simulink model "Energy"  (R2014a)
settings: Solver=ode45  StartTime=0.0  StopTime=10.0  RelTol=1e-3
undefined symbols (not defined in the file): nfs
settings Model: Creator=sadidsaze6  LastModifiedBy=sadidsaze6

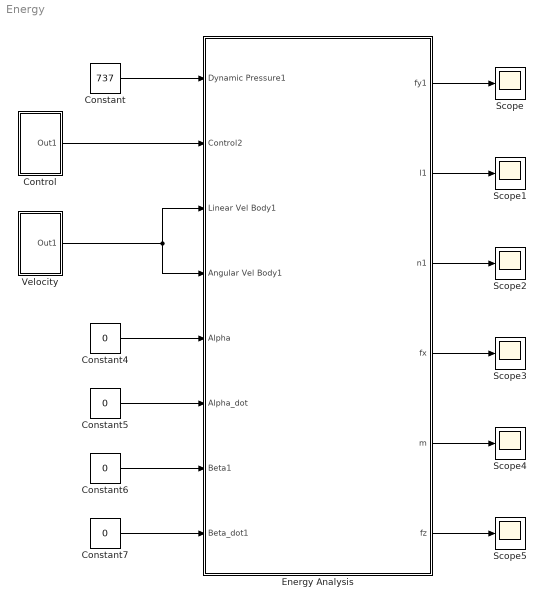
== system Energy ==
  Constant : Constant  Value=737
  Constant{4..7} (4 alike) : Constant  Value=0
  Control : Subsystem
  Energy Analysis : Subsystem  mask{ae=nfs}
      mask prompts: ae "Aero Coefficients"
  Scope{,1..5} (6 alike) : Scope
      Scope2 settings: SaveName=ScopeData2
      Scope3 settings: SaveName=ScopeData3
      Scope4 settings: SaveName=ScopeData4
      Scope5 settings: SaveName=ScopeData5
  Velocity : Subsystem
  wires:
  Constant4/1 -> Energy Analysis/5(Alpha)
  Constant/1 -> Energy Analysis/1(Dynamic Pressure1)
  Constant6/1 -> Energy Analysis/7(Beta1)
  Constant5/1 -> Energy Analysis/6(Alpha_dot)
  Constant7/1 -> Energy Analysis/8(Beta_dot1)
  Energy Analysis/2(l1) -> Scope1/1
  Energy Analysis/1(fy1) -> Scope/1
  Energy Analysis/3(n1) -> Scope2/1
  Energy Analysis/4(fx) -> Scope3/1
  Energy Analysis/5(m) -> Scope4/1
  Energy Analysis/6(fz) -> Scope5/1
  Control/1(Out1) -> Energy Analysis/2(Control2)
  Velocity/1(Out1) -> Energy Analysis/4(Angular Vel Body1), Energy Analysis/3(Linear Vel Body1)

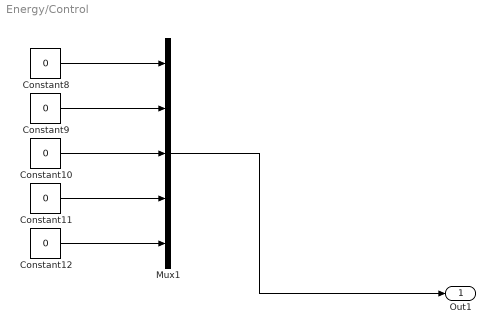
== system Energy/Control ==
  Constant{8..12} (5 alike) : Constant  Value=0
  Mux1 : Mux  Inputs=5
  Out1 : Outport
  wires:
  Mux1/1 -> Out1/1
  Constant10/1 -> Mux1/3
  Constant9/1 -> Mux1/2
  Constant8/1 -> Mux1/1
  Constant11/1 -> Mux1/4
  Constant12/1 -> Mux1/5

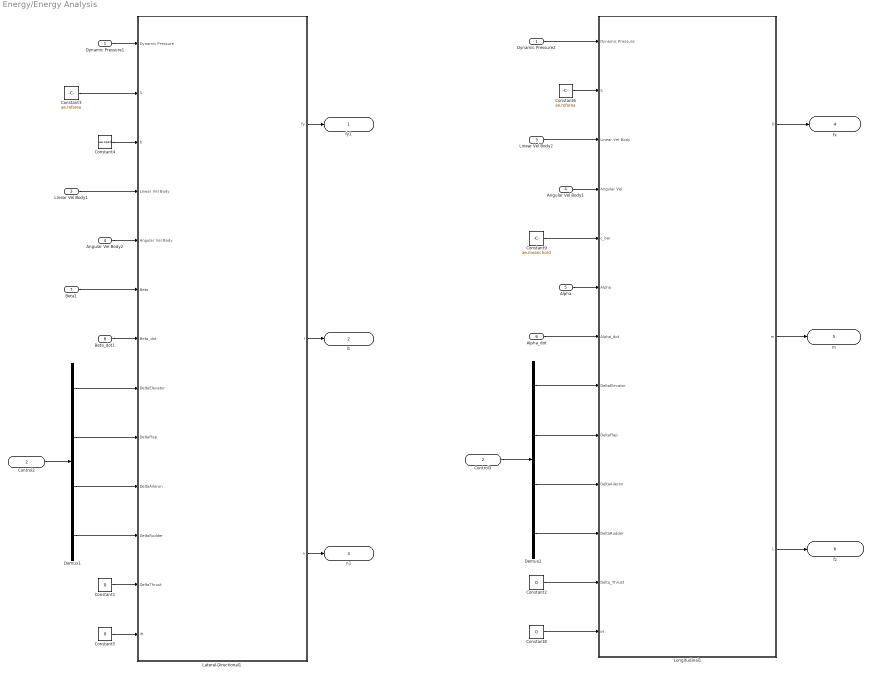
== system Energy/Energy Analysis ==
  Dynamic Pressure1 : Inport
  Control2 : Inport  Port=2
  Linear Vel Body1 : Inport  Port=3
  Angular Vel Body1 : Inport  Port=4
  Alpha : Inport  Port=5
  Alpha_dot : Inport  Port=6
  Beta1 : Inport  Port=7
  Beta_dot1 : Inport  Port=8
  Angular Vel Body2 : InportShadow  Port=4
  Constant{1..2,5,8} (4 alike) : Constant  Value=0
  Constant3 : Constant  Value=ae.refarea
  Constant4 : Constant  Value=ae.span
  Constant6 : Constant  Value=ae.refarea
  Constant9 : Constant  Value=ae.meanchord
  Control3 : InportShadow  Port=2
  Demux1 : Demux
  Demux2 : Demux
  Dynamic Pressure2 : InportShadow
  Lateral-Directional1 : Subsystem
  Linear Vel Body2 : InportShadow  Port=3
  Longitudinal1 : Subsystem
  fy1 : Outport
  l1 : Outport  Port=2
  n1 : Outport  Port=3
  fx : Outport  Port=4
  m : Outport  Port=5
  fz : Outport  Port=6
  wires:
  Lateral-Directional1/1(fy) -> fy1/1
  Lateral-Directional1/2(l) -> l1/1
  Lateral-Directional1/3(n) -> n1/1
  Longitudinal1/2(m) -> m/1
  Longitudinal1/1(D) -> fx/1
  Longitudinal1/3(L) -> fz/1
  Dynamic Pressure1/1 -> Lateral-Directional1/1(Dynamic Pressure)
  Constant3/1 -> Lateral-Directional1/2(S)
  Linear Vel Body1/1 -> Lateral-Directional1/4(Linear Vel Body)
  Angular Vel Body2/1 -> Lateral-Directional1/5(Angular Vel Body)
  Constant5/1 -> Lateral-Directional1/13(iH)
  Constant4/1 -> Lateral-Directional1/3(b)
  Beta1/1 -> Lateral-Directional1/6(Beta)
  Beta_dot1/1 -> Lateral-Directional1/7(Beta_dot)
  Demux1/1 -> Lateral-Directional1/8(DeltaElevator)
  Demux1/2 -> Lateral-Directional1/9(DeltaFlap)
  Demux1/4 -> Lateral-Directional1/11(DeltaRudder)
  Demux1/3 -> Lateral-Directional1/10(DeltaAileron)
  Constant1/1 -> Lateral-Directional1/12(DeltaThrust)
  Control2/1 -> Demux1/1
  Constant6/1 -> Longitudinal1/2(S)
  Alpha/1 -> Longitudinal1/6(Alpha)
  Angular Vel Body1/1 -> Longitudinal1/4(Angular Vel)
  Dynamic Pressure2/1 -> Longitudinal1/1(Dynamic Pressure)
  Linear Vel Body2/1 -> Longitudinal1/3(Linear Vel Body)
  Constant9/1 -> Longitudinal1/5(c_bar)
  Alpha_dot/1 -> Longitudinal1/7(Alpha_dot)
  Constant8/1 -> Longitudinal1/13(iH)
  Constant2/1 -> Longitudinal1/12(Delta_Thrust)
  Demux2/4 -> Longitudinal1/11(DeltaRudder)
  Demux2/2 -> Longitudinal1/9(DeltaFlap)
  Demux2/3 -> Longitudinal1/10(DeltaAileron)
  Demux2/1 -> Longitudinal1/8(DeltaElevator)
  Control3/1 -> Demux2/1

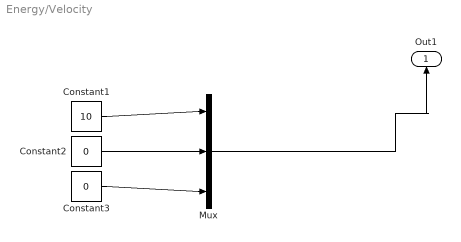
== system Energy/Velocity ==
  Constant1 : Constant  Value=10
  Constant2 : Constant  Value=0
  Constant3 : Constant  Value=0
  Mux : Mux  Inputs=3
  Out1 : Outport
  wires:
  Mux/1 -> Out1/1
  Constant2/1 -> Mux/2
  Constant1/1 -> Mux/1
  Constant3/1 -> Mux/3

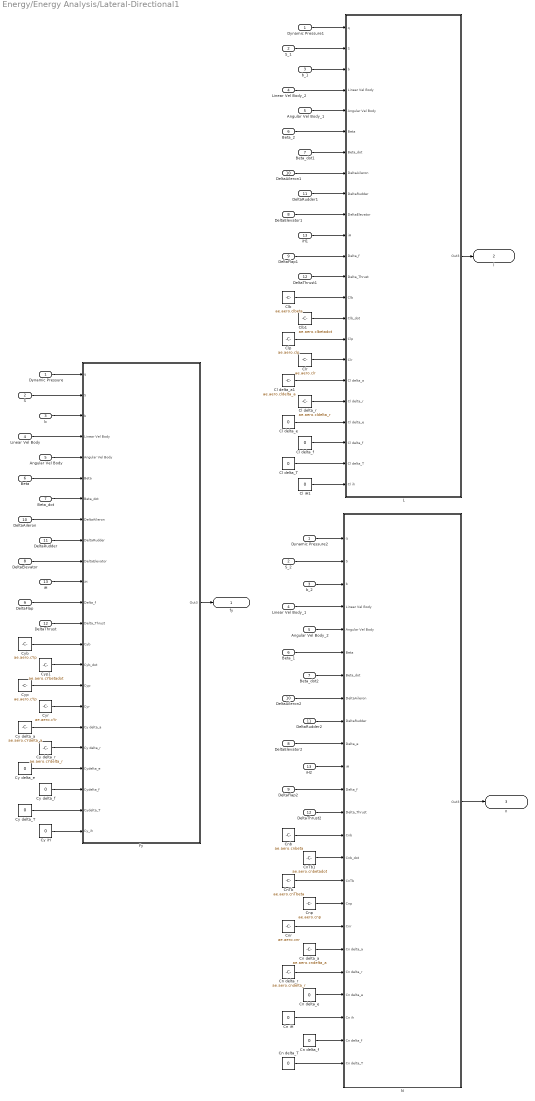
== system Energy/Energy Analysis/Lateral-Directional1 ==
  Dynamic Pressure : Inport
  S : Inport  Port=2
  b : Inport  Port=3
  Linear Vel Body : Inport  Port=4
  Angular Vel Body : Inport  Port=5
  Beta : Inport  Port=6
  Beta_dot : Inport  Port=7
  DeltaElevator : Inport  Port=8
  DeltaFlap : Inport  Port=9
  DeltaAileron : Inport  Port=10
  DeltaRudder : Inport  Port=11
  DeltaThrust : Inport  Port=12
  iH : Inport  Port=13
  Angular Vel Body_1 : InportShadow  Port=5
  Angular Vel Body_2 : InportShadow  Port=5
  Beta_1 : InportShadow  Port=6
  Beta_2 : InportShadow  Port=6
  Beta_dot1 : InportShadow  Port=7
  Beta_dot2 : InportShadow  Port=7
  Cl delta_T : Constant  Value=0
  Cl delta_a1 : Constant  Value=ae.aero.cldelta_a
  Cl delta_e : Constant  Value=0
  Cl delta_f : Constant  Value=0
  Cl delta_r : Constant  Value=ae.aero.cldelta_r
  Cl iH1 : Constant  Value=0
  Clb : Constant  Value=ae.aero.clbeta
  Clb1 : Constant  Value=ae.aero.clbetadot
  Clp : Constant  Value=ae.aero.clp
  Clr : Constant  Value=ae.aero.clr
  Cn delta_T : Constant  Value=0
  Cn delta_a : Constant  Value=ae.aero.cndelta_a
  Cn delta_e : Constant  Value=0
  Cn delta_f : Constant  Value=0
  Cn delta_r : Constant  Value=ae.aero.cndelta_r
  Cn iH : Constant  Value=0
  CnTb : Constant  Value=ae.aero.cnTbeta
  CnTb1 : Constant  Value=ae.aero.cnbetadot
  Cnb : Constant  Value=ae.aero.cnbeta
  Cnp : Constant  Value=ae.aero.cnp
  Cnr : Constant  Value=ae.aero.cnr
  Cy delta_T : Constant  Value=0
  Cy delta_a : Constant  Value=ae.aero.cYdelta_a
  Cy delta_e : Constant  Value=0
  Cy delta_f : Constant  Value=0
  Cy delta_r : Constant  Value=ae.aero.cYdelta_r
  Cy iH : Constant  Value=0
  Cyb : Constant  Value=ae.aero.cYp
  Cyp : Constant  Value=ae.aero.cYp
  Cyp1 : Constant  Value=ae.aero.cYbetadot
  Cyr : Constant  Value=ae.aero.cYr
  DeltaAileron1 : InportShadow  Port=10
  DeltaAileron2 : InportShadow  Port=10
  DeltaElevator1 : InportShadow  Port=8
  DeltaElevator2 : InportShadow  Port=8
  DeltaFlap1 : InportShadow  Port=9
  DeltaFlap2 : InportShadow  Port=9
  DeltaRudder1 : InportShadow  Port=11
  DeltaRudder2 : InportShadow  Port=11
  DeltaThrust1 : InportShadow  Port=12
  DeltaThrust2 : InportShadow  Port=12
  Dynamic Pressure1 : InportShadow
  Dynamic Pressure2 : InportShadow
  Fy : Subsystem
  L : Subsystem
  Linear Vel Body_1 : InportShadow  Port=4
  Linear Vel Body_2 : InportShadow  Port=4
  N : Subsystem
  S_1 : InportShadow  Port=2
  S_2 : InportShadow  Port=2
  b_1 : InportShadow  Port=3
  b_2 : InportShadow  Port=3
  iH1 : InportShadow  Port=13
  iH2 : InportShadow  Port=13
  fy : Outport
  l : Outport  Port=2
  n : Outport  Port=3
  wires:
  L/1(Out3) -> l/1
  N/1(Out3) -> n/1
  Fy/1(Out3) -> fy/1
  Dynamic Pressure/1 -> Fy/1(q)
  S/1 -> Fy/2(S)
  b/1 -> Fy/3(b)
  Linear Vel Body/1 -> Fy/4(Linear Vel Body)
  Angular Vel Body/1 -> Fy/5(Angular Vel Body)
  Beta/1 -> Fy/6(Beta)
  Beta_dot/1 -> Fy/7(Beta_dot)
  DeltaAileron/1 -> Fy/8(DeltaAileron)
  DeltaRudder/1 -> Fy/9(DeltaRudder)
  iH/1 -> Fy/11(iH)
  DeltaElevator/1 -> Fy/10(DeltaElevator)
  DeltaFlap/1 -> Fy/12(Delta_f)
  DeltaThrust/1 -> Fy/13(Delta_Thrust)
  DeltaRudder2/1 -> N/9(DeltaRudder)
  DeltaAileron2/1 -> N/8(DeltaAileron)
  Dynamic Pressure2/1 -> N/1(q)
  DeltaThrust2/1 -> N/13(Delta_Thrust)
  b_2/1 -> N/3(b)
  Angular Vel Body_2/1 -> N/5(Angular Vel Body)
  Linear Vel Body_1/1 -> N/4(Linear Vel Body)
  iH2/1 -> N/11(iH)
  Beta_dot2/1 -> N/7(Beta_dot)
  S_2/1 -> N/2(S)
  DeltaElevator2/1 -> N/10(Delta_e)
  DeltaFlap2/1 -> N/12(Delta_f)
  Beta_1/1 -> N/6(Beta)
  Cyb/1 -> Fy/14(Cyb)
  Cyp/1 -> Fy/16(Cyp)
  Cyr/1 -> Fy/17(Cyr)
  Cy delta_a/1 -> Fy/18(Cy delta_a)
  Cy delta_r/1 -> Fy/19(Cy delta_r)
  Cy delta_e/1 -> Fy/20(Cydelta_e)
  Cy delta_f/1 -> Fy/21(Cydelta_f)
  Cy delta_T/1 -> Fy/22(Cydelta_T)
  Cy iH/1 -> Fy/23(Cy_ih)
  Cnb/1 -> N/14(Cnb)
  Cnp/1 -> N/17(Cnp)
  Cn delta_T/1 -> N/24(Cn delta_T)
  CnTb/1 -> N/16(CnTb)
  Cn delta_a/1 -> N/19(Cn delta_a)
  Cn delta_e/1 -> N/21(Cn delta_e)
  Cn delta_r/1 -> N/20(Cn delta_r)
  Cn iH/1 -> N/22(Cn ih)
  Cn delta_f/1 -> N/23(Cn delta_f)
  Cnr/1 -> N/18(Cnr)
  Clb/1 -> L/14(Clb)
  Clp/1 -> L/16(Clp)
  Cl delta_a1/1 -> L/18(Cl delta_a)
  b_1/1 -> L/3(b)
  Dynamic Pressure1/1 -> L/1(q)
  Angular Vel Body_1/1 -> L/5(Angular Vel Body)
  iH1/1 -> L/11(iH)
  DeltaRudder1/1 -> L/9(DeltaRudder)
  DeltaThrust1/1 -> L/13(Delta_Thrust)
  Beta_dot1/1 -> L/7(Beta_dot)
  Beta_2/1 -> L/6(Beta)
  DeltaAileron1/1 -> L/8(DeltaAileron)
  DeltaFlap1/1 -> L/12(Delta_f)
  DeltaElevator1/1 -> L/10(DeltaElevator)
  Linear Vel Body_2/1 -> L/4(Linear Vel Body)
  S_1/1 -> L/2(S)
  Clr/1 -> L/17(Clr)
  Cl delta_e/1 -> L/20(Cl delta_e)
  Cl delta_T/1 -> L/22(Cl delta_T)
  Cl delta_f/1 -> L/21(Cl delta_f)
  Cl delta_r/1 -> L/19(Cl delta_r)
  Cl iH1/1 -> L/23(Cl ih)
  Clb1/1 -> L/15(Clb_dot)
  CnTb1/1 -> N/15(Cnb_dot)
  Cyp1/1 -> Fy/15(Cyb_dot)

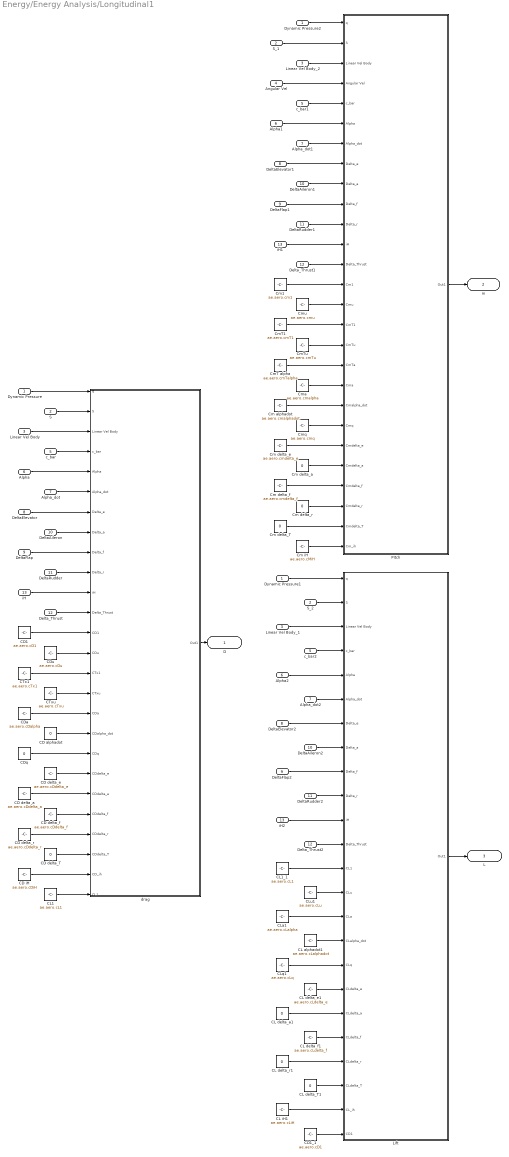
== system Energy/Energy Analysis/Longitudinal1 ==
  Dynamic Pressure : Inport
  S : Inport  Port=2
  Linear Vel Body : Inport  Port=3
  Angular Vel : Inport  Port=4
  c_bar : Inport  Port=5
  Alpha : Inport  Port=6
  Alpha_dot : Inport  Port=7
  DeltaElevator : Inport  Port=8
  DeltaFlap : Inport  Port=9
  DeltaAileron : Inport  Port=10
  DeltaRudder : Inport  Port=11
  Delta_Thrust : Inport  Port=12
  iH : Inport  Port=13
  Alpha1 : InportShadow  Port=6
  Alpha2 : InportShadow  Port=6
  Alpha_dot1 : InportShadow  Port=7
  Alpha_dot2 : InportShadow  Port=7
  CD alphadot : Constant  Value=0
  CD delta_T : Constant  Value=0
  CD delta_a : Constant  Value=ae.aero.cDdelta_a
  CD delta_e : Constant  Value=ae.aero.cDdelta_e
  CD delta_f : Constant  Value=ae.aero.cDdelta_f
  CD delta_r : Constant  Value=ae.aero.cDdelta_r
  CD iH : Constant  Value=ae.aero.cDiH
  CD1 : Constant  Value=ae.aero.cD1
  CD1_1 : Constant  Value=ae.aero.cD1
  CDa : Constant  Value=ae.aero.cDalpha
  CDq : Constant  Value=0
  CDu : Constant  Value=ae.aero.cDu
  CL alphadot1 : Constant  Value=ae.aero.cLalphadot
  CL delta_T1 : Constant  Value=0
  CL delta_a1 : Constant  Value=0
  CL delta_e1 : Constant  Value=ae.aero.cLdelta_e
  CL delta_f1 : Constant  Value=ae.aero.cLdelta_f
  CL delta_r1 : Constant  Value=0
  CL iH1 : Constant  Value=ae.aero.cLiH
  CL1 : Constant  Value=ae.aero.cL1
  CL1_1 : Constant  Value=ae.aero.cL1
  CLa1 : Constant  Value=ae.aero.cLalpha
  CLq1 : Constant  Value=ae.aero.cLq
  CLu1 : Constant  Value=ae.aero.cLu
  CTx1 : Constant  Value=ae.aero.cTx1
  CTxu : Constant  Value=ae.aero.cTxu
  Cm alphadot : Constant  Value=ae.aero.cmalphadot
  Cm delta_T : Constant  Value=0
  Cm delta_a : Constant  Value=0
  Cm delta_e : Constant  Value=ae.aero.cmdelta_e
  Cm delta_f : Constant  Value=ae.aero.cmdelta_f
  Cm delta_r : Constant  Value=0
  Cm iH : Constant  Value=ae.aero.cMiH
  Cm1 : Constant  Value=ae.aero.cm1
  CmT alpha : Constant  Value=ae.aero.cmTalpha
  CmT1 : Constant  Value=ae.aero.cmT1
  CmTu : Constant  Value=ae.aero.cmTu
  Cma : Constant  Value=ae.aero.cmalpha
  Cmq : Constant  Value=ae.aero.cmq
  Cmu : Constant  Value=ae.aero.cmu
  DeltaAileron1 : InportShadow  Port=10
  DeltaAileron2 : InportShadow  Port=10
  DeltaElevator1 : InportShadow  Port=8
  DeltaElevator2 : InportShadow  Port=8
  DeltaFlap1 : InportShadow  Port=9
  DeltaFlap2 : InportShadow  Port=9
  DeltaRudder1 : InportShadow  Port=11
  DeltaRudder2 : InportShadow  Port=11
  Delta_Thrust1 : InportShadow  Port=12
  Delta_Thrust2 : InportShadow  Port=12
  Dynamic Pressure1 : InportShadow
  Dynamic Pressure2 : InportShadow
  Lift : Subsystem
  Linear Vel Body_1 : InportShadow  Port=3
  Linear Vel Body_2 : InportShadow  Port=3
  Pitch : Subsystem
  S_1 : InportShadow  Port=2
  S_2 : InportShadow  Port=2
  c_bar1 : InportShadow  Port=5
  c_bar2 : InportShadow  Port=5
  drag : Subsystem
  iH1 : InportShadow  Port=13
  iH2 : InportShadow  Port=13
  D : Outport
  m : Outport  Port=2
  L : Outport  Port=3
  wires:
  DeltaRudder/1 -> drag/10(Delta_r)
  DeltaAileron/1 -> drag/8(Delta_a)
  CDa/1 -> drag/17(CDa)
  Alpha/1 -> drag/5(Alpha)
  CDu/1 -> drag/14(CDu)
  Alpha_dot/1 -> drag/6(Alpha_dot)
  drag/1(Out1) -> D/1
  Lift/1(Out1) -> L/1
  S/1 -> drag/2(S)
  Dynamic Pressure/1 -> drag/1(q)
  Linear Vel Body/1 -> drag/3(Linear Vel Body)
  Delta_Thrust/1 -> drag/12(Delta_Thrust)
  iH/1 -> drag/11(iH)
  CD delta_T/1 -> drag/24(CDdelta_T)
  DeltaElevator/1 -> drag/7(Delta_e)
  DeltaFlap/1 -> drag/9(Delta_f)
  Pitch/1(Out1) -> m/1
  c_bar/1 -> drag/4(c_bar)
  CD alphadot/1 -> drag/18(CDalpha_dot)
  CDq/1 -> drag/19(CDq)
  CD delta_e/1 -> drag/20(CDdelta_e)
  CD delta_a/1 -> drag/21(CDdelta_a)
  CD delta_f/1 -> drag/22(CDdelta_f)
  CD delta_r/1 -> drag/23(CDdelta_r)
  CD iH/1 -> drag/25(CD_ih)
  CTx1/1 -> drag/15(CTx1)
  CD1/1 -> drag/13(CD1)
  CTxu/1 -> drag/16(CTxu)
  DeltaRudder1/1 -> Pitch/11(Delta_r)
  DeltaAileron1/1 -> Pitch/9(Delta_a)
  Alpha1/1 -> Pitch/6(Alpha)
  Alpha_dot1/1 -> Pitch/7(Alpha_dot)
  S_1/1 -> Pitch/2(S)
  Dynamic Pressure2/1 -> Pitch/1(q)
  Linear Vel Body_2/1 -> Pitch/3(Linear Vel Body)
  Delta_Thrust1/1 -> Pitch/13(Delta_Thrust)
  iH1/1 -> Pitch/12(iH)
  DeltaElevator1/1 -> Pitch/8(Delta_e)
  DeltaFlap1/1 -> Pitch/10(Delta_f)
  S_2/1 -> Lift/2(S)
  Dynamic Pressure1/1 -> Lift/1(q)
  Linear Vel Body_1/1 -> Lift/3(Linear Vel Body)
  Delta_Thrust2/1 -> Lift/12(Delta_Thrust)
  c_bar2/1 -> Lift/4(c_bar)
  CL1/1 -> drag/26(CL1)
  iH2/1 -> Lift/11(iH)
  DeltaRudder2/1 -> Lift/10(Delta_r)
  DeltaFlap2/1 -> Lift/9(Delta_f)
  DeltaAileron2/1 -> Lift/8(Delta_a)
  DeltaElevator2/1 -> Lift/7(Delta_e)
  Alpha_dot2/1 -> Lift/6(Alpha_dot)
  Alpha2/1 -> Lift/5(Alpha)
  Angular Vel/1 -> Pitch/4(Angular Vel)
  c_bar1/1 -> Pitch/5(c_bar)
  CD1_1/1 -> Lift/24(CD1)
  CLa1/1 -> Lift/15(CLa)
  CLq1/1 -> Lift/17(CLq)
  CL delta_a1/1 -> Lift/19(CLdelta_a)
  CL delta_r1/1 -> Lift/21(CLdelta_r)
  CL iH1/1 -> Lift/23(CL_ih)
  CL delta_T1/1 -> Lift/22(CLdelta_T)
  CLu1/1 -> Lift/14(CLu)
  CL alphadot1/1 -> Lift/16(CLalpha_dot)
  CL delta_f1/1 -> Lift/20(CLdelta_f)
  CL delta_e1/1 -> Lift/18(CLdelta_e)
  CL1_1/1 -> Lift/13(CL1)
  CmT alpha/1 -> Pitch/18(CmTa)
  Cm alphadot/1 -> Pitch/20(Cmalpha_dot)
  Cm delta_e/1 -> Pitch/22(Cmdelta_e)
  Cm delta_f/1 -> Pitch/24(Cmdelta_f)
  Cm delta_T/1 -> Pitch/26(Cmdelta_T)
  CmT1/1 -> Pitch/16(CmT1)
  Cm1/1 -> Pitch/14(Cm1)
  CmTu/1 -> Pitch/17(CmTu)
  Cmq/1 -> Pitch/21(Cmq)
  Cm delta_a/1 -> Pitch/23(Cmdelta_a)
  Cm delta_r/1 -> Pitch/25(Cmdelta_r)
  Cmu/1 -> Pitch/15(Cmu)
  Cma/1 -> Pitch/19(Cma)
  Cm iH/1 -> Pitch/27(Cm_ih)

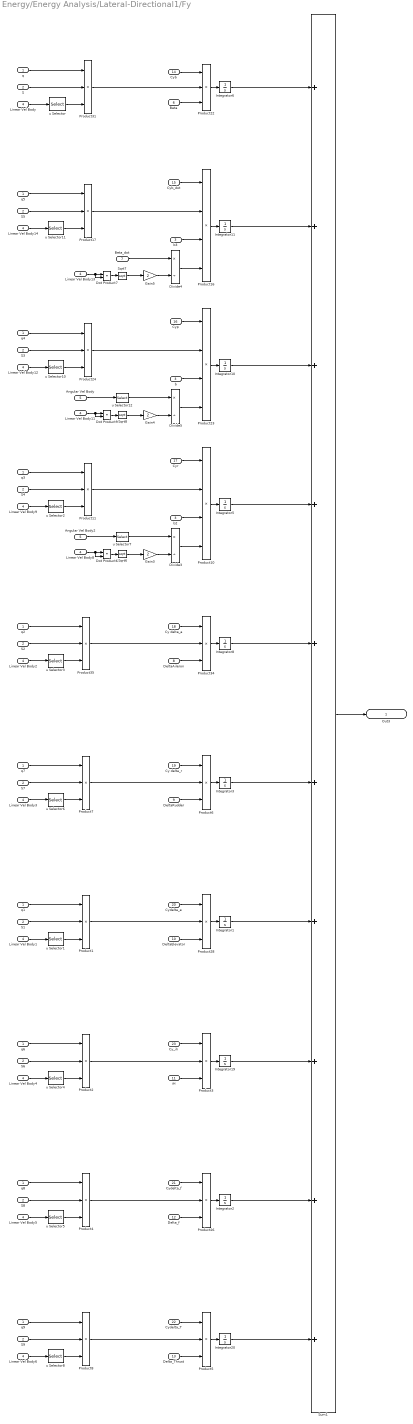
== system Energy/Energy Analysis/Lateral-Directional1/Fy ==
  q : Inport
  S : Inport  Port=2
  b : Inport  Port=3
  Linear Vel Body : Inport  Port=4
  Angular Vel Body : Inport  Port=5
  Beta : Inport  Port=6
  Beta_dot : Inport  Port=7
  DeltaAileron : Inport  Port=8
  DeltaRudder : Inport  Port=9
  DeltaElevator : Inport  Port=10
  iH : Inport  Port=11
  Delta_f : Inport  Port=12
  Delta_Thrust : Inport  Port=13
  Cyb : Inport  Port=14
  Cyb_dot : Inport  Port=15
  Cyp : Inport  Port=16
  Cyr : Inport  Port=17
  Cy delta_a : Inport  Port=18
  Cy delta_r : Inport  Port=19
  Cydelta_e : Inport  Port=20
  Cydelta_f : Inport  Port=21
  Cydelta_T : Inport  Port=22
  Cy_ih : Inport  Port=23
  Angular Vel Body2 : InportShadow  Port=5
  Divide3 : Product  Inputs=*/
  Divide4 : Product  Inputs=*/
  Divide5 : Product  Inputs=*/
  Dot Product6 : DotProduct  InputSameDT=on  OutDataTypeStr=Inherit: Inherit via internal rule
  Dot Product7 : DotProduct  InputSameDT=on  OutDataTypeStr=Inherit: Inherit via internal rule
  Dot Product9 : DotProduct  InputSameDT=on  OutDataTypeStr=Inherit: Inherit via internal rule
  Gain3 : Gain  Gain=2
  Gain4 : Gain  Gain=2
  Gain5 : Gain  Gain=2
  Integrator{1..3,5..6,8,10..11,19..20} (10 alike) : Integrator
  Linear Vel Body{1..6,8..9,11..14} (12 alike) : InportShadow  Port=4
  Product{1..8,11,17,22,24,26,28,31,34..35} (17 alike) : Product  Inputs=3
  Product10 : Product  Inputs=4
  Product16 : Product  Inputs=4
  Product23 : Product  Inputs=4
  S{1..9} (9 alike) : InportShadow  Port=2
  Sqrt6 : Sqrt  SaturateOnIntegerOverflow=on
  Sqrt7 : Sqrt  SaturateOnIntegerOverflow=on
  Sqrt8 : Sqrt  SaturateOnIntegerOverflow=on
  Sum1 : Sum  Inputs=++++++++++
  b2 : InportShadow  Port=3
  b3 : InportShadow  Port=3
  q{1..9} (9 alike) : InportShadow
  u Selector{,1..6,8,10..11} (10 alike) : Selector  InputPortWidth=3  Indices=[2]
  u Selector12 : Selector  InputPortWidth=3  Indices=[1]
  u Selector7 : Selector  InputPortWidth=3  Indices=[3]
  Out3 : Outport
  wires:
  Integrator11/1 -> Sum1/2
  q/1 -> Product31/1
  S/1 -> Product31/2
  u Selector/1 -> Product31/3
  Linear Vel Body/1 -> u Selector/1
  Cy delta_a/1 -> Product34/1
  Product35/1 -> Product34/2
  DeltaAileron/1 -> Product34/3
  Product34/1 -> Integrator8/1
  Integrator8/1 -> Sum1/5
  Product24/1 -> Product23/2
  Divide5/1 -> Product23/4
  Product23/1 -> Integrator10/1
  q4/1 -> Product24/1
  S3/1 -> Product24/2
  u Selector10/1 -> Product24/3
  Linear Vel Body12/1 -> u Selector10/1
  Sqrt8/1 -> Gain4/1
  u Selector12/1 -> Divide5/1
  Dot Product9/1 -> Sqrt8/1
  Linear Vel Body11/1 -> Dot Product9/2, Dot Product9/1
  Angular Vel Body/1 -> u Selector12/1
  Cyp/1 -> Product23/1
  Sum1/1 -> Out3/1
  Cyb/1 -> Product22/1
  Product31/1 -> Product22/2
  Beta/1 -> Product22/3
  Product22/1 -> Integrator6/1
  Integrator6/1 -> Sum1/1
  b/1 -> Product23/3
  Gain4/1 -> Divide5/2
  Product11/1 -> Product10/2
  Divide3/1 -> Product10/4
  Product10/1 -> Integrator5/1
  q3/1 -> Product11/1
  S4/1 -> Product11/2
  u Selector2/1 -> Product11/3
  Linear Vel Body9/1 -> u Selector2/1
  Sqrt6/1 -> Gain3/1
  u Selector7/1 -> Divide3/1
  Dot Product6/1 -> Sqrt6/1
  Linear Vel Body8/1 -> Dot Product6/1, Dot Product6/2
  Angular Vel Body2/1 -> u Selector7/1
  Cyr/1 -> Product10/1
  b2/1 -> Product10/3
  Gain3/1 -> Divide3/2
  Integrator10/1 -> Sum1/3
  Integrator5/1 -> Sum1/4
  Product17/1 -> Product16/2
  Divide4/1 -> Product16/4
  Product16/1 -> Integrator11/1
  q5/1 -> Product17/1
  S5/1 -> Product17/2
  u Selector11/1 -> Product17/3
  Linear Vel Body14/1 -> u Selector11/1
  Sqrt7/1 -> Gain5/1
  Beta_dot/1 -> Divide4/1
  Dot Product7/1 -> Sqrt7/1
  Linear Vel Body13/1 -> Dot Product7/1, Dot Product7/2
  Cyb_dot/1 -> Product16/1
  b3/1 -> Product16/3
  Gain5/1 -> Divide4/2
  Cydelta_T/1 -> Product5/1
  Product8/1 -> Product5/2
  Delta_Thrust/1 -> Product5/3
  Product5/1 -> Integrator20/1
  Cydelta_f/1 -> Product26/1
  Product4/1 -> Product26/2
  Delta_f/1 -> Product26/3
  Product26/1 -> Integrator2/1
  Cydelta_e/1 -> Product28/1
  Product1/1 -> Product28/2
  DeltaElevator/1 -> Product28/3
  Product28/1 -> Integrator1/1
  Cy_ih/1 -> Product3/1
  Product2/1 -> Product3/2
  iH/1 -> Product3/3
  Product3/1 -> Integrator19/1
  q2/1 -> Product35/1
  S2/1 -> Product35/2
  u Selector3/1 -> Product35/3
  Linear Vel Body2/1 -> u Selector3/1
  Cy delta_r/1 -> Product6/1
  Product7/1 -> Product6/2
  DeltaRudder/1 -> Product6/3
  Product6/1 -> Integrator3/1
  q7/1 -> Product7/1
  S7/1 -> Product7/2
  u Selector6/1 -> Product7/3
  Linear Vel Body3/1 -> u Selector6/1
  Integrator3/1 -> Sum1/6
  Integrator1/1 -> Sum1/7
  Integrator19/1 -> Sum1/8
  Integrator2/1 -> Sum1/9
  Integrator20/1 -> Sum1/10
  q1/1 -> Product1/1
  S1/1 -> Product1/2
  u Selector1/1 -> Product1/3
  Linear Vel Body1/1 -> u Selector1/1
  q6/1 -> Product2/1
  S6/1 -> Product2/2
  u Selector4/1 -> Product2/3
  Linear Vel Body4/1 -> u Selector4/1
  q8/1 -> Product4/1
  S8/1 -> Product4/2
  u Selector5/1 -> Product4/3
  Linear Vel Body5/1 -> u Selector5/1
  q9/1 -> Product8/1
  S9/1 -> Product8/2
  u Selector8/1 -> Product8/3
  Linear Vel Body6/1 -> u Selector8/1

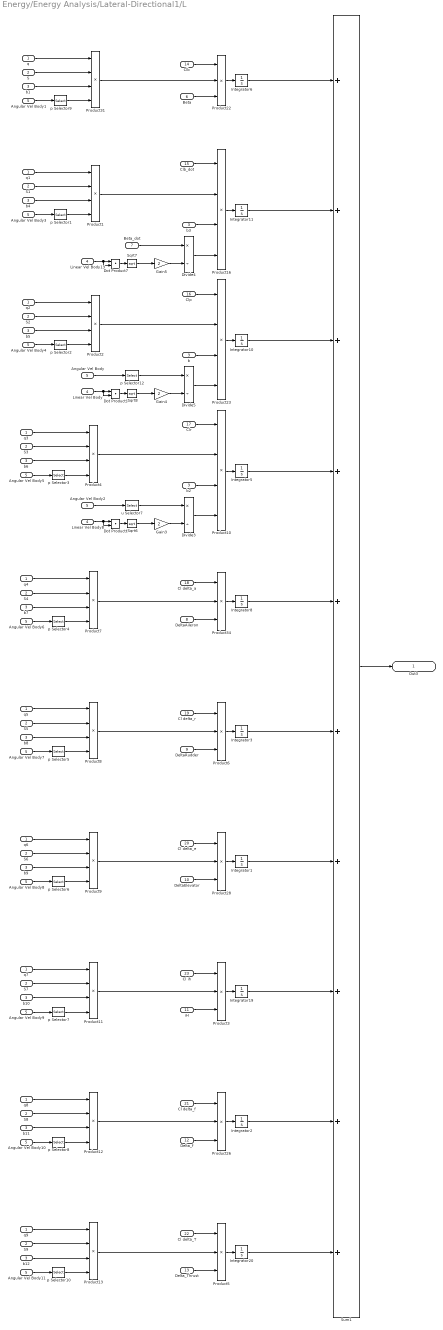
== system Energy/Energy Analysis/Lateral-Directional1/L ==
  q : Inport
  S : Inport  Port=2
  b : Inport  Port=3
  Linear Vel Body : Inport  Port=4
  Angular Vel Body : Inport  Port=5
  Beta : Inport  Port=6
  Beta_dot : Inport  Port=7
  DeltaAileron : Inport  Port=8
  DeltaRudder : Inport  Port=9
  DeltaElevator : Inport  Port=10
  iH : Inport  Port=11
  Delta_f : Inport  Port=12
  Delta_Thrust : Inport  Port=13
  Clb : Inport  Port=14
  Clb_dot : Inport  Port=15
  Clp : Inport  Port=16
  Clr : Inport  Port=17
  Cl delta_a : Inport  Port=18
  Cl delta_r : Inport  Port=19
  Cl delta_e : Inport  Port=20
  Cl delta_f : Inport  Port=21
  Cl delta_T : Inport  Port=22
  Cl ih : Inport  Port=23
  Angular Vel Body{1..11} (11 alike) : InportShadow  Port=5
  Divide3 : Product  Inputs=*/
  Divide4 : Product  Inputs=*/
  Divide5 : Product  Inputs=*/
  Dot Product6 : DotProduct  InputSameDT=on  OutDataTypeStr=Inherit: Inherit via internal rule
  Dot Product7 : DotProduct  InputSameDT=on  OutDataTypeStr=Inherit: Inherit via internal rule
  Dot Product9 : DotProduct  InputSameDT=on  OutDataTypeStr=Inherit: Inherit via internal rule
  Gain3 : Gain  Gain=2
  Gain4 : Gain  Gain=2
  Gain5 : Gain  Gain=2
  Integrator{1..3,5..6,8,10..11,19..20} (10 alike) : Integrator
  Linear Vel Body13 : InportShadow  Port=4
  Linear Vel Body8 : InportShadow  Port=4
  Product{1..2,4,7..13,16,23,31} (13 alike) : Product  Inputs=4
  Product{3,5..6,22,26,28,34} (7 alike) : Product  Inputs=3
  S{1..9} (9 alike) : InportShadow  Port=2
  Sqrt6 : Sqrt  SaturateOnIntegerOverflow=on
  Sqrt7 : Sqrt  SaturateOnIntegerOverflow=on
  Sqrt8 : Sqrt  SaturateOnIntegerOverflow=on
  Sum1 : Sum  Inputs=++++++++++
  b{1..12} (12 alike) : InportShadow  Port=3
  p Selector{1..10,12} (11 alike) : Selector  InputPortWidth=3  Indices=[1]
  q{1..9} (9 alike) : InportShadow
  u Selector7 : Selector  InputPortWidth=3  Indices=[3]
  Out3 : Outport
  wires:
  Integrator11/1 -> Sum1/2
  q/1 -> Product31/1
  S/1 -> Product31/2
  p Selector9/1 -> Product31/4
  Cl delta_a/1 -> Product34/1
  Product7/1 -> Product34/2
  DeltaAileron/1 -> Product34/3
  Product34/1 -> Integrator8/1
  Integrator8/1 -> Sum1/5
  Product2/1 -> Product23/2
  Divide5/1 -> Product23/4
  Product23/1 -> Integrator10/1
  Sqrt8/1 -> Gain4/1
  p Selector12/1 -> Divide5/1
  Dot Product9/1 -> Sqrt8/1
  Linear Vel Body/1 -> Dot Product9/2, Dot Product9/1
  Angular Vel Body/1 -> p Selector12/1
  Clp/1 -> Product23/1
  Sum1/1 -> Out3/1
  Clb/1 -> Product22/1
  Product31/1 -> Product22/2
  Beta/1 -> Product22/3
  Product22/1 -> Integrator6/1
  Integrator6/1 -> Sum1/1
  b/1 -> Product23/3
  Gain4/1 -> Divide5/2
  Product4/1 -> Product10/2
  Divide3/1 -> Product10/4
  Product10/1 -> Integrator5/1
  Sqrt6/1 -> Gain3/1
  u Selector7/1 -> Divide3/1
  Dot Product6/1 -> Sqrt6/1
  Linear Vel Body8/1 -> Dot Product6/1, Dot Product6/2
  Angular Vel Body2/1 -> u Selector7/1
  Clr/1 -> Product10/1
  b2/1 -> Product10/3
  Gain3/1 -> Divide3/2
  Integrator10/1 -> Sum1/3
  Integrator5/1 -> Sum1/4
  Product1/1 -> Product16/2
  Divide4/1 -> Product16/4
  Product16/1 -> Integrator11/1
  Sqrt7/1 -> Gain5/1
  Beta_dot/1 -> Divide4/1
  Dot Product7/1 -> Sqrt7/1
  Linear Vel Body13/1 -> Dot Product7/1, Dot Product7/2
  Clb_dot/1 -> Product16/1
  b3/1 -> Product16/3
  Gain5/1 -> Divide4/2
  Cl delta_T/1 -> Product5/1
  Product13/1 -> Product5/2
  Delta_Thrust/1 -> Product5/3
  Product5/1 -> Integrator20/1
  Cl delta_f/1 -> Product26/1
  Product12/1 -> Product26/2
  Delta_f/1 -> Product26/3
  Product26/1 -> Integrator2/1
  Cl delta_e/1 -> Product28/1
  Product9/1 -> Product28/2
  DeltaElevator/1 -> Product28/3
  Product28/1 -> Integrator1/1
  Cl ih/1 -> Product3/1
  Product11/1 -> Product3/2
  iH/1 -> Product3/3
  Product3/1 -> Integrator19/1
  Cl delta_r/1 -> Product6/1
  Product8/1 -> Product6/2
  DeltaRudder/1 -> Product6/3
  Product6/1 -> Integrator3/1
  Integrator3/1 -> Sum1/6
  Integrator1/1 -> Sum1/7
  Integrator19/1 -> Sum1/8
  Integrator2/1 -> Sum1/9
  Integrator20/1 -> Sum1/10
  Angular Vel Body1/1 -> p Selector9/1
  b1/1 -> Product31/3
  q1/1 -> Product1/1
  S1/1 -> Product1/2
  p Selector1/1 -> Product1/4
  Angular Vel Body3/1 -> p Selector1/1
  b4/1 -> Product1/3
  q2/1 -> Product2/1
  S2/1 -> Product2/2
  p Selector2/1 -> Product2/4
  Angular Vel Body4/1 -> p Selector2/1
  b5/1 -> Product2/3
  q3/1 -> Product4/1
  S3/1 -> Product4/2
  p Selector3/1 -> Product4/4
  Angular Vel Body5/1 -> p Selector3/1
  b6/1 -> Product4/3
  q4/1 -> Product7/1
  S4/1 -> Product7/2
  p Selector4/1 -> Product7/4
  Angular Vel Body6/1 -> p Selector4/1
  b7/1 -> Product7/3
  q5/1 -> Product8/1
  S5/1 -> Product8/2
  p Selector5/1 -> Product8/4
  Angular Vel Body7/1 -> p Selector5/1
  b8/1 -> Product8/3
  q6/1 -> Product9/1
  S6/1 -> Product9/2
  p Selector6/1 -> Product9/4
  Angular Vel Body8/1 -> p Selector6/1
  b9/1 -> Product9/3
  q7/1 -> Product11/1
  S7/1 -> Product11/2
  p Selector7/1 -> Product11/4
  Angular Vel Body9/1 -> p Selector7/1
  b10/1 -> Product11/3
  q8/1 -> Product12/1
  S8/1 -> Product12/2
  p Selector8/1 -> Product12/4
  Angular Vel Body10/1 -> p Selector8/1
  b11/1 -> Product12/3
  q9/1 -> Product13/1
  S9/1 -> Product13/2
  p Selector10/1 -> Product13/4
  Angular Vel Body11/1 -> p Selector10/1
  b12/1 -> Product13/3

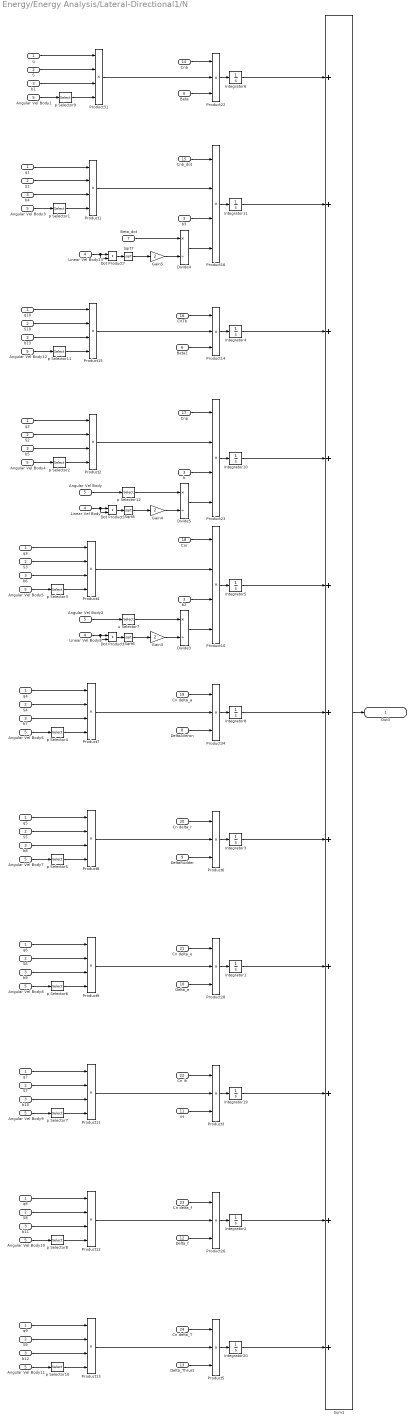
== system Energy/Energy Analysis/Lateral-Directional1/N ==
  q : Inport
  S : Inport  Port=2
  b : Inport  Port=3
  Linear Vel Body : Inport  Port=4
  Angular Vel Body : Inport  Port=5
  Beta : Inport  Port=6
  Beta_dot : Inport  Port=7
  DeltaAileron : Inport  Port=8
  DeltaRudder : Inport  Port=9
  Delta_e : Inport  Port=10
  iH : Inport  Port=11
  Delta_f : Inport  Port=12
  Delta_Thrust : Inport  Port=13
  Cnb : Inport  Port=14
  Cnb_dot : Inport  Port=15
  CnTb : Inport  Port=16
  Cnp : Inport  Port=17
  Cnr : Inport  Port=18
  Cn delta_a : Inport  Port=19
  Cn delta_r : Inport  Port=20
  Cn delta_e : Inport  Port=21
  Cn ih : Inport  Port=22
  Cn delta_f : Inport  Port=23
  Cn delta_T : Inport  Port=24
  Angular Vel Body{1..12} (12 alike) : InportShadow  Port=5
  Beta1 : InportShadow  Port=6
  Divide3 : Product  Inputs=*/
  Divide4 : Product  Inputs=*/
  Divide5 : Product  Inputs=*/
  Dot Product6 : DotProduct  InputSameDT=on  OutDataTypeStr=Inherit: Inherit via internal rule
  Dot Product7 : DotProduct  InputSameDT=on  OutDataTypeStr=Inherit: Inherit via internal rule
  Dot Product9 : DotProduct  InputSameDT=on  OutDataTypeStr=Inherit: Inherit via internal rule
  Gain3 : Gain  Gain=2
  Gain4 : Gain  Gain=2
  Gain5 : Gain  Gain=2
  Integrator{1..6,8,10..11,19..20} (11 alike) : Integrator
  Linear Vel Body13 : InportShadow  Port=4
  Linear Vel Body8 : InportShadow  Port=4
  Product{1..2,4,7..13,15..16,23,31} (14 alike) : Product  Inputs=4
  Product{3,5..6,14,22,26,28,34} (8 alike) : Product  Inputs=3
  S{1..10} (10 alike) : InportShadow  Port=2
  Sqrt6 : Sqrt  SaturateOnIntegerOverflow=on
  Sqrt7 : Sqrt  SaturateOnIntegerOverflow=on
  Sqrt8 : Sqrt  SaturateOnIntegerOverflow=on
  Sum1 : Sum  Inputs=+++++++++++
  b{1..13} (13 alike) : InportShadow  Port=3
  p Selector{1..12} (12 alike) : Selector  InputPortWidth=3  Indices=[1]
  q{1..10} (10 alike) : InportShadow
  u Selector7 : Selector  InputPortWidth=3  Indices=[3]
  Out3 : Outport
  wires:
  Integrator11/1 -> Sum1/2
  q/1 -> Product31/1
  S/1 -> Product31/2
  p Selector9/1 -> Product31/4
  Cn delta_a/1 -> Product34/1
  Product7/1 -> Product34/2
  DeltaAileron/1 -> Product34/3
  Product34/1 -> Integrator8/1
  Product2/1 -> Product23/2
  Divide5/1 -> Product23/4
  Product23/1 -> Integrator10/1
  Sqrt8/1 -> Gain4/1
  p Selector12/1 -> Divide5/1
  Dot Product9/1 -> Sqrt8/1
  Linear Vel Body/1 -> Dot Product9/2, Dot Product9/1
  Angular Vel Body/1 -> p Selector12/1
  Cnp/1 -> Product23/1
  Cnb/1 -> Product22/1
  Product31/1 -> Product22/2
  Beta/1 -> Product22/3
  Product22/1 -> Integrator6/1
  Integrator6/1 -> Sum1/1
  b/1 -> Product23/3
  Gain4/1 -> Divide5/2
  Product4/1 -> Product10/2
  Divide3/1 -> Product10/4
  Product10/1 -> Integrator5/1
  Sqrt6/1 -> Gain3/1
  u Selector7/1 -> Divide3/1
  Dot Product6/1 -> Sqrt6/1
  Linear Vel Body8/1 -> Dot Product6/1, Dot Product6/2
  Angular Vel Body2/1 -> u Selector7/1
  Cnr/1 -> Product10/1
  b2/1 -> Product10/3
  Gain3/1 -> Divide3/2
  Product1/1 -> Product16/2
  Divide4/1 -> Product16/4
  Product16/1 -> Integrator11/1
  Sqrt7/1 -> Gain5/1
  Beta_dot/1 -> Divide4/1
  Dot Product7/1 -> Sqrt7/1
  Linear Vel Body13/1 -> Dot Product7/1, Dot Product7/2
  Cnb_dot/1 -> Product16/1
  b3/1 -> Product16/3
  Gain5/1 -> Divide4/2
  Cn delta_T/1 -> Product5/1
  Product13/1 -> Product5/2
  Delta_Thrust/1 -> Product5/3
  Product5/1 -> Integrator20/1
  Cn delta_f/1 -> Product26/1
  Product12/1 -> Product26/2
  Delta_f/1 -> Product26/3
  Product26/1 -> Integrator2/1
  Cn delta_e/1 -> Product28/1
  Product9/1 -> Product28/2
  Delta_e/1 -> Product28/3
  Product28/1 -> Integrator1/1
  Cn ih/1 -> Product3/1
  Product11/1 -> Product3/2
  iH/1 -> Product3/3
  Product3/1 -> Integrator19/1
  Cn delta_r/1 -> Product6/1
  Product8/1 -> Product6/2
  DeltaRudder/1 -> Product6/3
  Product6/1 -> Integrator3/1
  Angular Vel Body1/1 -> p Selector9/1
  b1/1 -> Product31/3
  q1/1 -> Product1/1
  S1/1 -> Product1/2
  p Selector1/1 -> Product1/4
  Angular Vel Body3/1 -> p Selector1/1
  b4/1 -> Product1/3
  q2/1 -> Product2/1
  S2/1 -> Product2/2
  p Selector2/1 -> Product2/4
  Angular Vel Body4/1 -> p Selector2/1
  b5/1 -> Product2/3
  q3/1 -> Product4/1
  S3/1 -> Product4/2
  p Selector3/1 -> Product4/4
  Angular Vel Body5/1 -> p Selector3/1
  b6/1 -> Product4/3
  q4/1 -> Product7/1
  S4/1 -> Product7/2
  p Selector4/1 -> Product7/4
  Angular Vel Body6/1 -> p Selector4/1
  b7/1 -> Product7/3
  q5/1 -> Product8/1
  S5/1 -> Product8/2
  p Selector5/1 -> Product8/4
  Angular Vel Body7/1 -> p Selector5/1
  b8/1 -> Product8/3
  q6/1 -> Product9/1
  S6/1 -> Product9/2
  p Selector6/1 -> Product9/4
  Angular Vel Body8/1 -> p Selector6/1
  b9/1 -> Product9/3
  q7/1 -> Product11/1
  S7/1 -> Product11/2
  p Selector7/1 -> Product11/4
  Angular Vel Body9/1 -> p Selector7/1
  b10/1 -> Product11/3
  q8/1 -> Product12/1
  S8/1 -> Product12/2
  p Selector8/1 -> Product12/4
  Angular Vel Body10/1 -> p Selector8/1
  b11/1 -> Product12/3
  q9/1 -> Product13/1
  S9/1 -> Product13/2
  p Selector10/1 -> Product13/4
  Angular Vel Body11/1 -> p Selector10/1
  b12/1 -> Product13/3
  q10/1 -> Product15/1
  S10/1 -> Product15/2
  p Selector11/1 -> Product15/4
  CnTb/1 -> Product14/1
  Product15/1 -> Product14/2
  Beta1/1 -> Product14/3
  Product14/1 -> Integrator4/1
  Angular Vel Body12/1 -> p Selector11/1
  b13/1 -> Product15/3
  Integrator20/1 -> Sum1/11
  Integrator2/1 -> Sum1/10
  Integrator19/1 -> Sum1/9
  Integrator1/1 -> Sum1/8
  Integrator3/1 -> Sum1/7
  Integrator8/1 -> Sum1/6
  Integrator5/1 -> Sum1/5
  Integrator10/1 -> Sum1/4
  Integrator4/1 -> Sum1/3
  Sum1/1 -> Out3/1

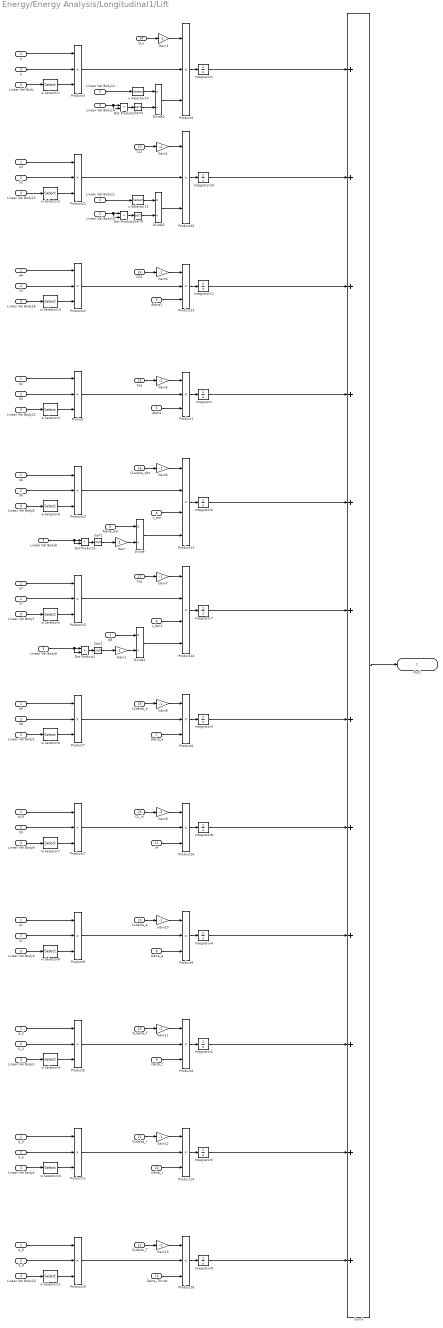
== system Energy/Energy Analysis/Longitudinal1/Lift ==
  q : Inport
  S : Inport  Port=2
  Linear Vel Body : Inport  Port=3
  c_bar : Inport  Port=4
  Alpha : Inport  Port=5
  Alpha_dot : Inport  Port=6
  Delta_e : Inport  Port=7
  Delta_a : Inport  Port=8
  Delta_f : Inport  Port=9
  Delta_r : Inport  Port=10
  iH : Inport  Port=11
  Delta_Thrust : Inport  Port=12
  CL1 : Inport  Port=13
  CLu : Inport  Port=14
  CLa : Inport  Port=15
  CLalpha_dot : Inport  Port=16
  CLq : Inport  Port=17
  CLdelta_e : Inport  Port=18
  CLdelta_a : Inport  Port=19
  CLdelta_f : Inport  Port=20
  CLdelta_r : Inport  Port=21
  CLdelta_T : Inport  Port=22
  CL_ih : Inport  Port=23
  CD1 : Inport  Port=24
  Alpha1 : InportShadow  Port=5
  Divide{,1..3} (4 alike) : Product  Inputs=*/
  Dot Product{1..4} (4 alike) : DotProduct  InputSameDT=on  OutDataTypeStr=Inherit: Inherit via internal rule
  Gain : Gain  Gain=2
  Gain1 : Gain  Gain=2
  Gain{3..13} (11 alike) : Gain  Gain=-1
  Gain2 : Gain  Gain=-2
  Integrator{,1..11} (12 alike) : Integrator
  Linear Vel Body{1..16,22} (17 alike) : InportShadow  Port=3
  Product{,1..11,13,15..23} (22 alike) : Product  Inputs=3
  Product12 : Product  Inputs=4
  Product14 : Product  Inputs=4
  S{1..3,5..9} (8 alike) : InportShadow  Port=2
  S_2 : InportShadow  Port=2
  S_5 : InportShadow  Port=2
  S_9 : InportShadow  Port=2
  Sqrt{1..4} (4 alike) : Sqrt  SaturateOnIntegerOverflow=on
  Sum3 : Sum  Inputs=++++++++++++
  c_bar1 : InportShadow  Port=4
  q{1..4,6..10} (9 alike) : InportShadow
  q_2 : InportShadow
  q_5 : InportShadow
  q_9 : InportShadow
  u Selector10 : Selector  InputPortWidth=3  Indices=[1]
  u Selector12 : Selector  InputPortWidth=3  Indices=[1]
  w Selector{1..11,13} (12 alike) : Selector  InputPortWidth=3  Indices=[3]
  Out1 : Outport
  wires:
  Integrator1/1 -> Sum3/1
  CLu/1 -> Gain3/1
  Product3/1 -> Product2/2
  Divide2/1 -> Product2/3
  Product2/1 -> Integrator1/1
  Integrator10/1 -> Sum3/2
  q/1 -> Product3/1
  S/1 -> Product3/2
  Sum3/1 -> Out1/1
  w Selector1/1 -> Product3/3
  Linear Vel Body/1 -> w Selector1/1
  Sqrt3/1 -> Divide2/2
  u Selector10/1 -> Divide2/1
  Dot Product2/1 -> Sqrt3/1
  Linear Vel Body14/1 -> Dot Product2/1, Dot Product2/2
  Linear Vel Body12/1 -> u Selector10/1
  CL1/1 -> Gain2/1
  Product21/1 -> Product20/2
  Divide3/1 -> Product20/3
  Product20/1 -> Integrator10/1
  q3/1 -> Product21/1
  S2/1 -> Product21/2
  w Selector2/1 -> Product21/3
  Linear Vel Body13/1 -> w Selector2/1
  Sqrt4/1 -> Divide3/2
  u Selector12/1 -> Divide3/1
  Dot Product4/1 -> Sqrt4/1
  Linear Vel Body15/1 -> Dot Product4/2, Dot Product4/1
  Linear Vel Body11/1 -> u Selector12/1
  Gain2/1 -> Product20/1
  Integrator6/1 -> Sum3/5
  Integrator3/1 -> Sum3/7
  Integrator4/1 -> Sum3/9
  Integrator2/1 -> Sum3/10
  Integrator5/1 -> Sum3/11
  CLdelta_T/1 -> Gain13/1
  Product19/1 -> Product18/2
  Delta_Thrust/1 -> Product18/3
  Product18/1 -> Integrator9/1
  q_9/1 -> Product19/1
  S_9/1 -> Product19/2
  w Selector11/1 -> Product19/3
  Linear Vel Body10/1 -> w Selector11/1
  Integrator9/1 -> Sum3/12
  CLdelta_r/1 -> Gain12/1
  Product11/1 -> Product10/2
  Delta_r/1 -> Product10/3
  Product10/1 -> Integrator5/1
  q_5/1 -> Product11/1
  S_5/1 -> Product11/2
  w Selector10/1 -> Product11/3
  Linear Vel Body4/1 -> w Selector10/1
  CLdelta_f/1 -> Gain11/1
  Product5/1 -> Product4/2
  Delta_f/1 -> Product4/3
  Product4/1 -> Integrator2/1
  q_2/1 -> Product5/1
  S_2/1 -> Product5/2
  w Selector9/1 -> Product5/3
  Linear Vel Body1/1 -> w Selector9/1
  Alpha/1 -> Product1/3
  CLa/1 -> Gain5/1
  Product/1 -> Product1/2
  Product1/1 -> Integrator/1
  q2/1 -> Product/1
  S5/1 -> Product/2
  Linear Vel Body22/1 -> w Selector3/1
  w Selector3/1 -> Product/3
  CLdelta_e/1 -> Gain8/1
  Product7/1 -> Product6/2
  Delta_e/1 -> Product6/3
  Product6/1 -> Integrator3/1
  q9/1 -> Product7/1
  S8/1 -> Product7/2
  w Selector6/1 -> Product7/3
  Linear Vel Body2/1 -> w Selector6/1
  CLdelta_a/1 -> Gain10/1
  Product9/1 -> Product8/2
  Delta_a/1 -> Product8/3
  Product8/1 -> Integrator4/1
  q1/1 -> Product9/1
  S1/1 -> Product9/2
  w Selector8/1 -> Product9/3
  Linear Vel Body3/1 -> w Selector8/1
  CLalpha_dot/1 -> Gain6/1
  Product13/1 -> Product12/2
  c_bar/1 -> Product12/3
  Product12/1 -> Integrator6/1
  q6/1 -> Product13/1
  S6/1 -> Product13/2
  w Selector4/1 -> Product13/3
  Linear Vel Body5/1 -> w Selector4/1
  Gain/1 -> Divide/2
  Alpha_dot/1 -> Divide/1
  Divide/1 -> Product12/4
  Dot Product3/1 -> Sqrt1/1
  Linear Vel Body6/1 -> Dot Product3/1, Dot Product3/2
  Sqrt1/1 -> Gain/1
  CLq/1 -> Gain7/1
  Product15/1 -> Product14/2
  c_bar1/1 -> Product14/3
  Product14/1 -> Integrator7/1
  q7/1 -> Product15/1
  S7/1 -> Product15/2
  w Selector5/1 -> Product15/3
  Linear Vel Body7/1 -> w Selector5/1
  Gain1/1 -> Divide1/2
  q8/1 -> Divide1/1
  Divide1/1 -> Product14/4
  Dot Product1/1 -> Sqrt2/1
  Linear Vel Body8/1 -> Dot Product1/2, Dot Product1/1
  Sqrt2/1 -> Gain1/1
  CL_ih/1 -> Gain9/1
  Product17/1 -> Product16/2
  iH/1 -> Product16/3
  Product16/1 -> Integrator8/1
  q10/1 -> Product17/1
  S9/1 -> Product17/2
  w Selector7/1 -> Product17/3
  Linear Vel Body9/1 -> w Selector7/1
  Integrator8/1 -> Sum3/8
  Integrator/1 -> Sum3/4
  Integrator7/1 -> Sum3/6
  Alpha1/1 -> Product23/3
  CD1/1 -> Gain4/1
  Product22/1 -> Product23/2
  Product23/1 -> Integrator11/1
  q4/1 -> Product22/1
  S3/1 -> Product22/2
  Linear Vel Body16/1 -> w Selector13/1
  w Selector13/1 -> Product22/3
  Integrator11/1 -> Sum3/3
  Gain3/1 -> Product2/1
  Gain4/1 -> Product23/1
  Gain5/1 -> Product1/1
  Gain6/1 -> Product12/1
  Gain7/1 -> Product14/1
  Gain8/1 -> Product6/1
  Gain9/1 -> Product16/1
  Gain10/1 -> Product8/1
  Gain11/1 -> Product4/1
  Gain12/1 -> Product10/1
  Gain13/1 -> Product18/1

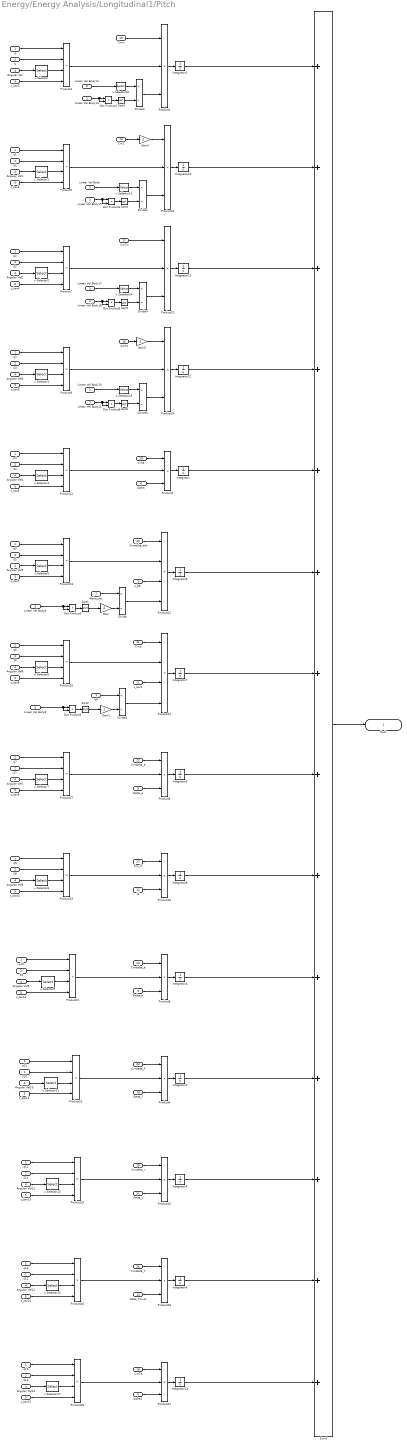
== system Energy/Energy Analysis/Longitudinal1/Pitch ==
  q : Inport
  S : Inport  Port=2
  Linear Vel Body : Inport  Port=3
  Angular Vel : Inport  Port=4
  c_bar : Inport  Port=5
  Alpha : Inport  Port=6
  Alpha_dot : Inport  Port=7
  Delta_e : Inport  Port=8
  Delta_a : Inport  Port=9
  Delta_f : Inport  Port=10
  Delta_r : Inport  Port=11
  iH : Inport  Port=12
  Delta_Thrust : Inport  Port=13
  Cm1 : Inport  Port=14
  Cmu : Inport  Port=15
  CmT1 : Inport  Port=16
  CmTu : Inport  Port=17
  CmTa : Inport  Port=18
  Cma : Inport  Port=19
  Cmalpha_dot : Inport  Port=20
  Cmq : Inport  Port=21
  Cmdelta_e : Inport  Port=22
  Cmdelta_a : Inport  Port=23
  Cmdelta_f : Inport  Port=24
  Cmdelta_r : Inport  Port=25
  Cmdelta_T : Inport  Port=26
  Cm_ih : Inport  Port=27
  Alpha1 : InportShadow  Port=6
  Angular Vel{1..13} (13 alike) : InportShadow  Port=4
  Divide{,1..5} (6 alike) : Product  Inputs=*/
  Dot Product{1..6} (6 alike) : DotProduct  InputSameDT=on  OutDataTypeStr=Inherit: Inherit via internal rule
  Gain{,1..3} (4 alike) : Gain  Gain=2
  Integrator{,1..13} (14 alike) : Integrator
  Linear Vel Body{6,8,12,14..15,17..19,21} (9 alike) : InportShadow  Port=3
  Product{1..2,4,6,8,10,16,18,20,22,24,27} (12 alike) : Product  Inputs=3
  Product{3,5,7,9,11..15,17,19,21,23,25..26,28} (16 alike) : Product  Inputs=4
  S{1..13} (13 alike) : InportShadow  Port=2
  Sqrt{1..6} (6 alike) : Sqrt  SaturateOnIntegerOverflow=on
  Sum3 : Sum  Inputs=++++++++++++++
  c_bar{1..15} (15 alike) : InportShadow  Port=5
  q{1..14} (14 alike) : InportShadow
  u Selector{,1..9,11,13,15,17} (14 alike) : Selector  InputPortWidth=3  Indices=[2]
  u Selector{10,12,14,16} (4 alike) : Selector  InputPortWidth=3  Indices=[1]
  Out1 : Outport
  wires:
  Integrator7/1 -> Sum3/7
  Integrator12/1 -> Sum3/4
  Gain3/1 -> Product24/1
  Linear Vel Body19/1 -> u Selector16/1
  Linear Vel Body21/1 -> Dot Product6/1, Dot Product6/2
  Dot Product6/1 -> Sqrt6/1
  u Selector16/1 -> Divide5/1
  Sqrt6/1 -> Divide5/2
  Product24/1 -> Integrator12/1
  Divide5/1 -> Product24/3
  Product9/1 -> Product24/2
  CmT1/1 -> Gain3/1
  Integrator11/1 -> Sum3/3
  Linear Vel Body17/1 -> u Selector14/1
  Linear Vel Body18/1 -> Dot Product5/2, Dot Product5/1
  Dot Product5/1 -> Sqrt5/1
  u Selector14/1 -> Divide4/1
  Sqrt5/1 -> Divide4/2
  Product22/1 -> Integrator11/1
  Divide4/1 -> Product22/3
  Product7/1 -> Product22/2
  CmTu/1 -> Product22/1
  Gain2/1 -> Product20/1
  Linear Vel Body/1 -> u Selector12/1
  Linear Vel Body15/1 -> Dot Product4/1, Dot Product4/2
  Dot Product4/1 -> Sqrt4/1
  u Selector12/1 -> Divide3/1
  Sqrt4/1 -> Divide3/2
  Product20/1 -> Integrator10/1
  Divide3/1 -> Product20/3
  Product5/1 -> Product20/2
  Cm1/1 -> Gain2/1
  Integrator/1 -> Sum3/5
  Integrator8/1 -> Sum3/9
  Product16/1 -> Integrator8/1
  iH/1 -> Product16/3
  Product19/1 -> Product16/2
  Cm_ih/1 -> Product16/1
  Sqrt2/1 -> Gain1/1
  Linear Vel Body8/1 -> Dot Product1/1, Dot Product1/2
  Dot Product1/1 -> Sqrt2/1
  Divide1/1 -> Product14/4
  q8/1 -> Divide1/1
  Gain1/1 -> Divide1/2
  Product14/1 -> Integrator7/1
  c_bar1/1 -> Product14/3
  Product15/1 -> Product14/2
  Cmq/1 -> Product14/1
  Sqrt1/1 -> Gain/1
  Linear Vel Body6/1 -> Dot Product3/2, Dot Product3/1
  Dot Product3/1 -> Sqrt1/1
  Divide/1 -> Product12/4
  Alpha_dot/1 -> Divide/1
  Gain/1 -> Divide/2
  Product12/1 -> Integrator6/1
  c_bar/1 -> Product12/3
  Product13/1 -> Product12/2
  Cmalpha_dot/1 -> Product12/1
  Product8/1 -> Integrator4/1
  Delta_a/1 -> Product8/3
  Product21/1 -> Product8/2
  Cmdelta_a/1 -> Product8/1
  Product6/1 -> Integrator3/1
  Delta_e/1 -> Product6/3
  Product17/1 -> Product6/2
  Cmdelta_e/1 -> Product6/1
  Product1/1 -> Integrator/1
  Product11/1 -> Product1/2
  Cma/1 -> Product1/1
  Alpha/1 -> Product1/3
  Product4/1 -> Integrator2/1
  Delta_f/1 -> Product4/3
  Product23/1 -> Product4/2
  Cmdelta_f/1 -> Product4/1
  Product10/1 -> Integrator5/1
  Delta_r/1 -> Product10/3
  Product25/1 -> Product10/2
  Cmdelta_r/1 -> Product10/1
  Integrator9/1 -> Sum3/13
  Product18/1 -> Integrator9/1
  Delta_Thrust/1 -> Product18/3
  Product26/1 -> Product18/2
  Cmdelta_T/1 -> Product18/1
  Integrator5/1 -> Sum3/12
  Integrator2/1 -> Sum3/11
  Integrator4/1 -> Sum3/10
  Integrator3/1 -> Sum3/8
  Integrator6/1 -> Sum3/6
  Linear Vel Body12/1 -> u Selector10/1
  Linear Vel Body14/1 -> Dot Product2/2, Dot Product2/1
  Dot Product2/1 -> Sqrt3/1
  u Selector10/1 -> Divide2/1
  Sqrt3/1 -> Divide2/2
  Angular Vel/1 -> u Selector/1
  u Selector/1 -> Product3/3
  Sum3/1 -> Out1/1
  S/1 -> Product3/2
  q/1 -> Product3/1
  Integrator10/1 -> Sum3/2
  Product2/1 -> Integrator1/1
  Divide2/1 -> Product2/3
  Product3/1 -> Product2/2
  Integrator1/1 -> Sum3/1
  CmTa/1 -> Product27/1
  Product28/1 -> Product27/2
  Product27/1 -> Integrator13/1
  Alpha1/1 -> Product27/3
  Integrator13/1 -> Sum3/14
  c_bar2/1 -> Product3/4
  Angular Vel1/1 -> u Selector1/1
  u Selector1/1 -> Product5/3
  S1/1 -> Product5/2
  q1/1 -> Product5/1
  c_bar3/1 -> Product5/4
  Angular Vel2/1 -> u Selector2/1
  u Selector2/1 -> Product7/3
  S2/1 -> Product7/2
  q2/1 -> Product7/1
  c_bar4/1 -> Product7/4
  Angular Vel3/1 -> u Selector3/1
  u Selector3/1 -> Product9/3
  S3/1 -> Product9/2
  q3/1 -> Product9/1
  c_bar5/1 -> Product9/4
  Angular Vel4/1 -> u Selector4/1
  u Selector4/1 -> Product11/3
  S4/1 -> Product11/2
  q4/1 -> Product11/1
  c_bar6/1 -> Product11/4
  Angular Vel5/1 -> u Selector5/1
  u Selector5/1 -> Product13/3
  S5/1 -> Product13/2
  q5/1 -> Product13/1
  c_bar7/1 -> Product13/4
  Angular Vel6/1 -> u Selector6/1
  u Selector6/1 -> Product15/3
  S6/1 -> Product15/2
  q6/1 -> Product15/1
  c_bar8/1 -> Product15/4
  Angular Vel7/1 -> u Selector7/1
  u Selector7/1 -> Product17/3
  S7/1 -> Product17/2
  q7/1 -> Product17/1
  c_bar9/1 -> Product17/4
  Angular Vel8/1 -> u Selector8/1
  u Selector8/1 -> Product19/3
  S8/1 -> Product19/2
  q9/1 -> Product19/1
  c_bar10/1 -> Product19/4
  Angular Vel9/1 -> u Selector9/1
  u Selector9/1 -> Product21/3
  S9/1 -> Product21/2
  q10/1 -> Product21/1
  c_bar11/1 -> Product21/4
  Angular Vel10/1 -> u Selector11/1
  u Selector11/1 -> Product23/3
  S10/1 -> Product23/2
  q11/1 -> Product23/1
  c_bar12/1 -> Product23/4
  Angular Vel11/1 -> u Selector13/1
  u Selector13/1 -> Product25/3
  S11/1 -> Product25/2
  q12/1 -> Product25/1
  c_bar13/1 -> Product25/4
  Angular Vel12/1 -> u Selector15/1
  u Selector15/1 -> Product26/3
  S12/1 -> Product26/2
  q13/1 -> Product26/1
  c_bar14/1 -> Product26/4
  Angular Vel13/1 -> u Selector17/1
  u Selector17/1 -> Product28/3
  S13/1 -> Product28/2
  q14/1 -> Product28/1
  c_bar15/1 -> Product28/4
  Cmu/1 -> Product2/1

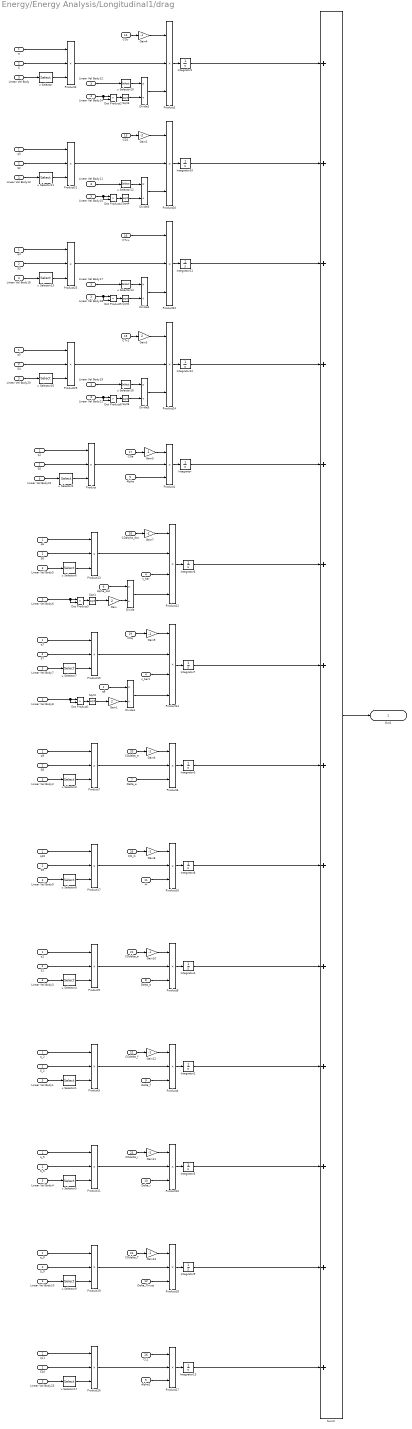
== system Energy/Energy Analysis/Longitudinal1/drag ==
  q : Inport
  S : Inport  Port=2
  Linear Vel Body : Inport  Port=3
  c_bar : Inport  Port=4
  Alpha : Inport  Port=5
  Alpha_dot : Inport  Port=6
  Delta_e : Inport  Port=7
  Delta_a : Inport  Port=8
  Delta_f : Inport  Port=9
  Delta_r : Inport  Port=10
  iH : Inport  Port=11
  Delta_Thrust : Inport  Port=12
  CD1 : Inport  Port=13
  CDu : Inport  Port=14
  CTx1 : Inport  Port=15
  CTxu : Inport  Port=16
  CDa : Inport  Port=17
  CDalpha_dot : Inport  Port=18
  CDq : Inport  Port=19
  CDdelta_e : Inport  Port=20
  CDdelta_a : Inport  Port=21
  CDdelta_f : Inport  Port=22
  CDdelta_r : Inport  Port=23
  CDdelta_T : Inport  Port=24
  CD_ih : Inport  Port=25
  CL1 : Inport  Port=26
  Alpha1 : InportShadow  Port=5
  Divide{,1..5} (6 alike) : Product  Inputs=*/
  Dot Product{1..6} (6 alike) : DotProduct  InputSameDT=on  OutDataTypeStr=Inherit: Inherit via internal rule
  Gain : Gain  Gain=2
  Gain1 : Gain  Gain=2
  Gain{4..13} (10 alike) : Gain  Gain=-1
  Gain2 : Gain  Gain=-2
  Gain3 : Gain  Gain=2
  Integrator{,1..13} (14 alike) : Integrator
  Linear Vel Body{1..23} (23 alike) : InportShadow  Port=3
  Product{,1..11,13,15..27} (26 alike) : Product  Inputs=3
  Product12 : Product  Inputs=4
  Product14 : Product  Inputs=4
  S{1..10} (10 alike) : InportShadow  Port=2
  S_2 : InportShadow  Port=2
  S_5 : InportShadow  Port=2
  S_9 : InportShadow  Port=2
  Sqrt{1..6} (6 alike) : Sqrt  SaturateOnIntegerOverflow=on
  Sum3 : Sum  Inputs=++++++++++++++
  c_bar1 : InportShadow  Port=4
  q{1..11} (11 alike) : InportShadow
  q_2 : InportShadow
  q_5 : InportShadow
  q_9 : InportShadow
  u Selector{,1..17} (18 alike) : Selector  InputPortWidth=3  Indices=[1]
  Out1 : Outport
  wires:
  Integrator1/1 -> Sum3/1
  CDu/1 -> Gain4/1
  Product3/1 -> Product2/2
  Divide2/1 -> Product2/3
  Product2/1 -> Integrator1/1
  Integrator10/1 -> Sum3/2
  q/1 -> Product3/1
  S/1 -> Product3/2
  Sum3/1 -> Out1/1
  u Selector/1 -> Product3/3
  Linear Vel Body/1 -> u Selector/1
  Sqrt3/1 -> Divide2/2
  u Selector10/1 -> Divide2/1
  Dot Product2/1 -> Sqrt3/1
  Linear Vel Body14/1 -> Dot Product2/1, Dot Product2/2
  Linear Vel Body12/1 -> u Selector10/1
  Integrator6/1 -> Sum3/6
  Integrator3/1 -> Sum3/8
  Integrator4/1 -> Sum3/10
  Integrator2/1 -> Sum3/11
  Integrator5/1 -> Sum3/12
  CDdelta_T/1 -> Gain13/1
  Product19/1 -> Product18/2
  Delta_Thrust/1 -> Product18/3
  Product18/1 -> Integrator9/1
  q_9/1 -> Product19/1
  S_9/1 -> Product19/2
  u Selector9/1 -> Product19/3
  Linear Vel Body10/1 -> u Selector9/1
  Integrator9/1 -> Sum3/13
  CDdelta_r/1 -> Gain11/1
  Product11/1 -> Product10/2
  Delta_r/1 -> Product10/3
  Product10/1 -> Integrator5/1
  q_5/1 -> Product11/1
  S_5/1 -> Product11/2
  u Selector5/1 -> Product11/3
  Linear Vel Body4/1 -> u Selector5/1
  CDdelta_f/1 -> Gain12/1
  Product5/1 -> Product4/2
  Delta_f/1 -> Product4/3
  Product4/1 -> Integrator2/1
  q_2/1 -> Product5/1
  S_2/1 -> Product5/2
  u Selector1/1 -> Product5/3
  Linear Vel Body1/1 -> u Selector1/1
  Alpha/1 -> Product1/3
  CDa/1 -> Gain5/1
  Product/1 -> Product1/2
  Product1/1 -> Integrator/1
  q2/1 -> Product/1
  S5/1 -> Product/2
  Linear Vel Body22/1 -> u Selector2/1
  u Selector2/1 -> Product/3
  CDdelta_e/1 -> Gain6/1
  Product7/1 -> Product6/2
  Delta_e/1 -> Product6/3
  Product6/1 -> Integrator3/1
  q9/1 -> Product7/1
  S8/1 -> Product7/2
  u Selector3/1 -> Product7/3
  Linear Vel Body2/1 -> u Selector3/1
  CDdelta_a/1 -> Gain10/1
  Product9/1 -> Product8/2
  Delta_a/1 -> Product8/3
  Product8/1 -> Integrator4/1
  q1/1 -> Product9/1
  S1/1 -> Product9/2
  u Selector4/1 -> Product9/3
  Linear Vel Body3/1 -> u Selector4/1
  CDalpha_dot/1 -> Gain7/1
  Product13/1 -> Product12/2
  c_bar/1 -> Product12/3
  Product12/1 -> Integrator6/1
  q6/1 -> Product13/1
  S6/1 -> Product13/2
  u Selector6/1 -> Product13/3
  Linear Vel Body5/1 -> u Selector6/1
  Gain/1 -> Divide/2
  Alpha_dot/1 -> Divide/1
  Divide/1 -> Product12/4
  Dot Product3/1 -> Sqrt1/1
  Linear Vel Body6/1 -> Dot Product3/1, Dot Product3/2
  Sqrt1/1 -> Gain/1
  CDq/1 -> Gain9/1
  Product15/1 -> Product14/2
  c_bar1/1 -> Product14/3
  Product14/1 -> Integrator7/1
  q7/1 -> Product15/1
  S7/1 -> Product15/2
  u Selector7/1 -> Product15/3
  Linear Vel Body7/1 -> u Selector7/1
  Gain1/1 -> Divide1/2
  q8/1 -> Divide1/1
  Divide1/1 -> Product14/4
  Dot Product1/1 -> Sqrt2/1
  Linear Vel Body8/1 -> Dot Product1/2, Dot Product1/1
  Sqrt2/1 -> Gain1/1
  CD_ih/1 -> Gain8/1
  Product17/1 -> Product16/2
  iH/1 -> Product16/3
  Product16/1 -> Integrator8/1
  q10/1 -> Product17/1
  S9/1 -> Product17/2
  u Selector8/1 -> Product17/3
  Linear Vel Body9/1 -> u Selector8/1
  Integrator8/1 -> Sum3/9
  Integrator/1 -> Sum3/5
  CD1/1 -> Gain2/1
  Product21/1 -> Product20/2
  Divide3/1 -> Product20/3
  Product20/1 -> Integrator10/1
  q3/1 -> Product21/1
  S2/1 -> Product21/2
  u Selector11/1 -> Product21/3
  Linear Vel Body13/1 -> u Selector11/1
  Sqrt4/1 -> Divide3/2
  u Selector12/1 -> Divide3/1
  Dot Product4/1 -> Sqrt4/1
  Linear Vel Body15/1 -> Dot Product4/2, Dot Product4/1
  Linear Vel Body11/1 -> u Selector12/1
  Gain2/1 -> Product20/1
  CTxu/1 -> Product22/1
  Product23/1 -> Product22/2
  Divide4/1 -> Product22/3
  Product22/1 -> Integrator11/1
  q4/1 -> Product23/1
  S3/1 -> Product23/2
  u Selector13/1 -> Product23/3
  Linear Vel Body16/1 -> u Selector13/1
  Sqrt5/1 -> Divide4/2
  u Selector14/1 -> Divide4/1
  Dot Product5/1 -> Sqrt5/1
  Linear Vel Body18/1 -> Dot Product5/1, Dot Product5/2
  Linear Vel Body17/1 -> u Selector14/1
  Integrator11/1 -> Sum3/3
  CTx1/1 -> Gain3/1
  Product25/1 -> Product24/2
  Divide5/1 -> Product24/3
  Product24/1 -> Integrator12/1
  q5/1 -> Product25/1
  S4/1 -> Product25/2
  u Selector15/1 -> Product25/3
  Linear Vel Body20/1 -> u Selector15/1
  Sqrt6/1 -> Divide5/2
  u Selector16/1 -> Divide5/1
  Dot Product6/1 -> Sqrt6/1
  Linear Vel Body21/1 -> Dot Product6/2, Dot Product6/1
  Linear Vel Body19/1 -> u Selector16/1
  Gain3/1 -> Product24/1
  Integrator12/1 -> Sum3/4
  Integrator7/1 -> Sum3/7
  Alpha1/1 -> Product27/3
  CL1/1 -> Product27/1
  Product26/1 -> Product27/2
  Product27/1 -> Integrator13/1
  q11/1 -> Product26/1
  S10/1 -> Product26/2
  Linear Vel Body23/1 -> u Selector17/1
  u Selector17/1 -> Product26/3
  Integrator13/1 -> Sum3/14
  Gain4/1 -> Product2/1
  Gain5/1 -> Product1/1
  Gain6/1 -> Product6/1
  Gain7/1 -> Product12/1
  Gain9/1 -> Product14/1
  Gain8/1 -> Product16/1
  Gain10/1 -> Product8/1
  Gain12/1 -> Product4/1
  Gain11/1 -> Product10/1
  Gain13/1 -> Product18/1
